simulink model "CodeGenValidation"  (R2018b)
settings: Solver=FixedStepDiscrete  StartTime=0.0  StopTime=60  FixedStep=MdlTS  RelTol=1e-3  EnableMultiTasking=on
undefined symbols (not defined in the file or in its folder): sigbuilder_block
settings Model: DataDictionary=CodeGenPlantData.sldd  Creator=BRAUL  LastModifiedBy=BRAUL
settings OptimizationCC: DefaultParameterBehavior=Inlined  UseFloatMulNetSlope=on  UseSpecifiedMinMax=on  InlineInvariantSignals=on  PassReuseOutputArgsAs=Individual arguments  ZeroExternalMemoryAtStartup=off  ZeroInternalMemoryAtStartup=off  NoFixptDivByZeroProtection=on  EfficientFloat2IntCast=on  LifeSpan=inf  MaxStackSize=64  OptimizeBlockOrder=speed  DifferentSizesBufferReuse=on
settings DebuggingCC: MergeDetectMultiDrivingBlocksExec=none  ParameterTunabilityLossMsg=error
settings HardwareCC: ProdBitPerPointer=32  ProdBitPerSizeT=32  ProdBitPerPtrDiffT=32  ProdLargestAtomicInteger=Long  ProdLargestAtomicFloat=Double  ProdWordSize=32  ProdLongLongMode=on  ProdHWDeviceType=ARM Compatible->ARM Cortex
settings ModelReferenceCC: ModelReferenceNumInstancesAllowed=Single  PropagateSignalLabelsOutOfModel=off
settings SFSimCC: MATLABDynamicMemAlloc=off
settings RTWCC: SystemTargetFile=ert.tlc  HardwareBoard=STM32 Nucleo F411RE  TemplateMakefile=ert_default_tmf  GenerateReport=on  Toolchain=GNU Tools for ARM Embedded Processors  BuildConfiguration=Faster Runs  IncludeHyperlinkInReport=on  LaunchReport=on  CodeExecutionProfiling=on  GenerateTraceInfo=on  GenerateTraceReport=on  GenerateTraceReportSl=on  GenerateTraceReportSf=on  GenerateTraceReportEml=on
settings CodeAppCC: ForceParamTrailComments=on  IgnoreCustomStorageClasses=off  OperatorAnnotations=on  SimulinkDataObjDesc=on  SFDataObjDesc=on  InsertBlockDesc=on
settings ERTTargetCC: CombineSignalStateStructs=on  SuppressErrorStatus=on  SupportNonFinite=off  SupportComplex=off

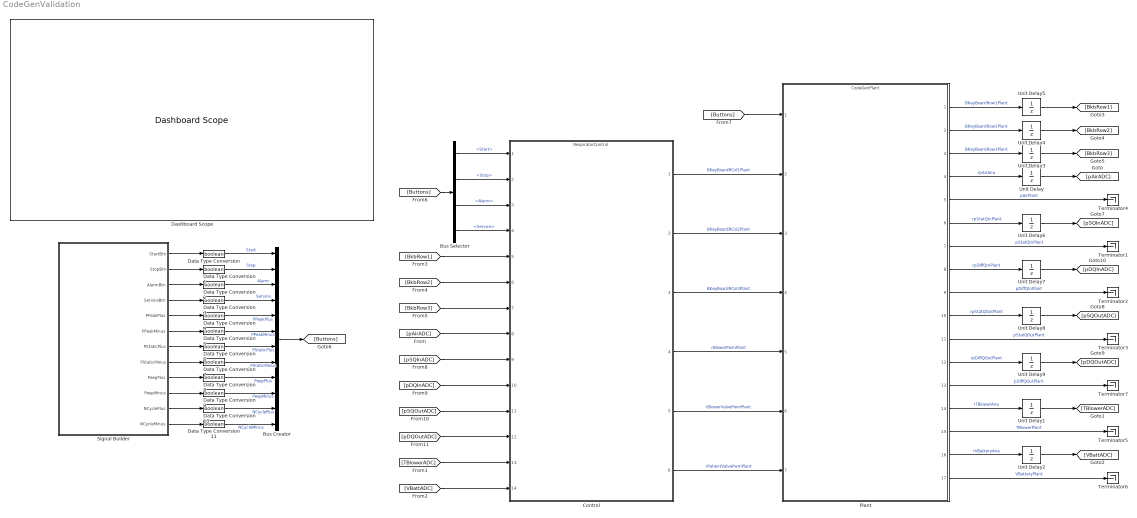
== system CodeGenValidation ==
  Bus Creator : BusCreator  Inputs=12  OutDataTypeStr=Bus: UserButtons
  Bus Selector : BusSelector  OutputSignals=Start,Stop,Alarm,Service
  Control : ModelReference  ModelNameDialog=RespiratorControl.slx  SimulationMode=Processor-in-the-loop (PIL)  ModelReferenceVersion=1.242
  Dashboard Scope : DashboardScope  WebBlockId=143  Ymin=0  Ymax=500
  Data Type Conversion{,1..11} (12 alike) : DataTypeConversion  OutDataTypeStr=boolean
  Plant : ModelReference  ModelNameDialog=CodeGenPlant.slx  SimulationMode=Normal  ModelReferenceVersion=1.68
  Signal Builder : Subsystem  Tag=STV Subsys  LoadFcn=sigbuilder_block('load');  StartFcn=sigbuilder_block('start');  StopFcn=sigbuilder_block('stop');  ClipboardFcn=sigbuilder_block('clipboard');  mask(Sigbuilder block){tuvar=[0:10]}
      mask help: Simulink:masks:SigbuilderBlock_MD
      mask init:
      | if ~strcmp(get_param(bdroot(gcbh),'SimulationStatus'),'stopped') tuvar = sigbuilder_block('maskInit'); end
      settings: CopyFcn=sigbuilder_block('copy');  DeleteFcn=sigbuilder_block('delete');  ModelCloseFcn=sigbuilder_block('modelClose');  PreSaveFcn=sigbuilder_block('preSave');  PauseFcn=sigbuilder_block('pause');  ContinueFcn=sigbuilder_block('continue');  NameChangeFcn=sigbuilder_block('namechange');  OpenFcn=sigbuilder_block('open',[6 0 1428 711.75 ]);  CloseFcn=sigbuilder_block('close');
      mask Display: plot(0, 0, 100, 100,[2, 2, 32, 32, 2], [68, 8, 8, 68, 68],[32, 2], [38, 38], [32, 19, 2],[53, 60, 44], [32, 17, 17, 2],[16, 16, 31, 31]);txt = getActiveGroup(gcbh);text(2, 100, txt,'verticalAlignment', 'top');
  Terminator{1..7} (7 alike) : Terminator
  Unit Delay{,2..5} (5 alike) : UnitDelay  SampleTime=-1
  Unit Delay{1,6..9} (5 alike) : UnitDelay  InitialCondition=0.7619  SampleTime=-1
  wires:
  Control/4 -> Plant/5  "rBlowerPwmPlant"
  Control/5 -> Plant/6  "rBlowerValvePwmPlant"
  Control/6 -> Plant/7  "rPatientValvePwmPlant"
  Plant/4 -> Unit Delay/1  "rpAirAna"
  Unit Delay/1 -> [pAirADC]
  [pAirADC] -> Control/8
  Bus Selector/1 -> Control/1  "<Start>"
  Bus Selector/2 -> Control/2  "<Stop>"
  Bus Selector/3 -> Control/3  "<Alarm>"
  Bus Selector/4 -> Control/4  "<Service>"
  Plant/5 -> Terminator4/1  "pAirPlant"
  Plant/15 -> Terminator5/1  "TBlowerPlant"
  Plant/17 -> Terminator6/1  "VBatteryPlant"
  Unit Delay1/1 -> [TBlowerADC]
  Plant/14 -> Unit Delay1/1  "rTBlowerAna"
  Plant/16 -> Unit Delay2/1  "rVBatteryAna"
  Unit Delay2/1 -> [VBattADC]
  [VBattADC] -> Control/14
  [TBlowerADC] -> Control/13
  Control/3 -> Plant/4  "BKeyBoardRCol3Plant"
  Control/2 -> Plant/3  "BKeyBoardRCol2Plant"
  Control/1 -> Plant/2  "BKeyBoardRCol1Plant"
  Plant/1 -> Unit Delay5/1  "BKeyBoardRow1Plant"
  Plant/2 -> Unit Delay4/1  "BKeyBoardRow2Plant"
  Plant/3 -> Unit Delay3/1  "BKeyBoardRow3Plant"
  Unit Delay5/1 -> [BkbRow1]
  Unit Delay4/1 -> [BkbRow2]
  Unit Delay3/1 -> [BkbRow3]
  [BkbRow1] -> Control/5
  [BkbRow2] -> Control/6
  [BkbRow3] -> Control/7
  Signal Builder/1(StartBtn) -> Data Type Conversion/1
  Signal Builder/2(StopBtn) -> Data Type Conversion1/1
  Signal Builder/3(AlarmBtn) -> Data Type Conversion2/1
  Signal Builder/4(ServiceBtn) -> Data Type Conversion3/1
  Signal Builder/5(PPeakPlus) -> Data Type Conversion4/1
  Signal Builder/6(PPeakMinus) -> Data Type Conversion5/1
  Signal Builder/7(PStaticPlus) -> Data Type Conversion6/1
  Signal Builder/8(PStaticMinus) -> Data Type Conversion7/1
  Signal Builder/9(PeepPlus) -> Data Type Conversion8/1
  Signal Builder/10(PeepMinus) -> Data Type Conversion9/1
  Signal Builder/11(NCyclePlus) -> Data Type Conversion10/1
  Signal Builder/12(NCycleMinus) -> Data Type Conversion11/1
  Bus Creator/1 -> [Buttons]
  [Buttons] -> Bus Selector/1
  [Buttons] -> Plant/1
  Data Type Conversion/1 -> Bus Creator/1  "Start"
  Data Type Conversion1/1 -> Bus Creator/2  "Stop"
  Data Type Conversion2/1 -> Bus Creator/3  "Alarm"
  Data Type Conversion3/1 -> Bus Creator/4  "Service"
  Data Type Conversion4/1 -> Bus Creator/5  "PPeakPlus"
  Data Type Conversion5/1 -> Bus Creator/6  "PPeakMinus"
  Data Type Conversion6/1 -> Bus Creator/7  "PStaticPlus"
  Data Type Conversion7/1 -> Bus Creator/8  "PStaticMinus"
  Data Type Conversion8/1 -> Bus Creator/9  "PeepPlus"
  Data Type Conversion9/1 -> Bus Creator/10  "PeepMinus"
  Data Type Conversion10/1 -> Bus Creator/11  "NCyclePlus"
  Data Type Conversion11/1 -> Bus Creator/12  "NCycleMinus"
  Plant/7 -> Terminator1/1  "pStatQInPlant"
  Plant/9 -> Terminator2/1  "pDiffQInPlant"
  Plant/11 -> Terminator3/1  "pStatQOutPlant"
  Plant/13 -> Terminator7/1  "pDiffQOutPlant"
  Plant/6 -> Unit Delay6/1  "rpStatQInPlant"
  Plant/10 -> Unit Delay8/1  "rpStatQOutPlant"
  Plant/8 -> Unit Delay7/1  "rpDiffQInPlant"
  Plant/12 -> Unit Delay9/1  "rpDiffQOutPlant"
  Unit Delay6/1 -> [pSQInADC]
  Unit Delay8/1 -> [pSQOutADC]
  Unit Delay9/1 -> [pDQOutADC]
  Unit Delay7/1 -> [pDQInADC]
  [pSQInADC] -> Control/9
  [pDQInADC] -> Control/10
  [pSQOutADC] -> Control/11
  [pDQOutADC] -> Control/12

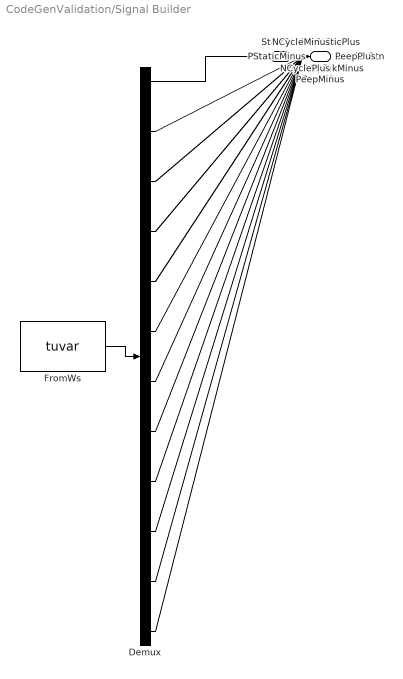
== system CodeGenValidation/Signal Builder ==
  Demux : Demux  Tag=STV Demux  Outputs=12
  FromWs : FromWorkspace  Tag=STV FromWs  VariableName=tuvar  SampleTime=0
      SigBuilderData=|
      | common.afterFinalStr = 'Extrapolate'
      | common.sampleTime = 0
      | dataSet.timeRange = [0 60]
      | dataSet.name = 'Group 1'
      | sbobj.Groups.Name = 'Group 1'
      | sbobj.Groups.Signals(1).Name = 'StartBtn'
      | sbobj.Groups.Signals(1).XData = [0 2 2 2.113 2.113 3 3 3.3 3.3 5.4 5.4 5.65 5.65 14 16 18 20 22 24 26 28 30 32 34 36 38 40 42 44 46 48 50 52 54 56 59.4 59.4 60]
      | sbobj.Groups.Signals(1).YData = [0 0 1 1 0 0 1 1 0 0 1 1 0 0 0 0 0 0 0 0 0 0 0 0 0 0 0 0 0 0 0 0 0 0 0 0 1 1]
      | sbobj.Groups.Signals(2).Name = 'StopBtn'
      | sbobj.Groups.Signals(2).XData = [0 0.75 0.75 1.1 1.1 6 8 10 12 14 16 18 20 22 24 26 28 30 32 34 36 38 40 42 44 46 48 56.05 56.05 56.07 56.07 57.1 57.1 57.65 57.65 58 60]
      | sbobj.Groups.Signals(2).YData = [0 0 1 1 0 0 0 0 0 0 0 0 0 0 0 0 0 0 0 0 0 0 0 0 0 0 0 0 1 1 0 0 1 1 0 0 0]
      | sbobj.Groups.Signals(3).Name = 'AlarmBtn'
      | sbobj.Groups.Signals(3).XData = [0 2 4 6 8 10 12 14 16 18 20 22 24 26 26 26.3 26.3 30 32 34 36 38 40 43.75 43.75 44 44 46 48 50 52 54 54 54.1 54.1 58 60]
      | sbobj.Groups.Signals(3).YData = [0 0 0 0 0 0 0 0 0 0 0 0 0 0 1 1 0 0 0 0 0 0 0 0 1 1 0 0 0 0 0 0 1 1 0 0 0]
      | sbobj.Groups.Signals(4).Name = 'ServiceBtn'
      | sbobj.Groups.Signals(4).XData = [0 2 4 6 8 10 12 14 16 18 20 22 24 26 28 30 32 34 36 38 40 40.7 40.7 41.2 41.2 46 48 50 52 54 56 58 60]
      | sbobj.Groups.Signals(4).YData = [0 0 0 0 0 0 0 0 0 0 0 0 0 0 0 0 0 0 0 0 0 0 1 1 0 0 0 0 0 0 0 0 0]
      | sbobj.Groups.Signals(5).Name = 'PPeakPlus'
      | sbobj.Groups.Signals(5).XData = [0 10.75 10.75 11 11 11.8 11.8 12.15 12.15 13.05 13.05 13.3 13.3 14.1 14.1 14.45 14.45 18 20 22 24 26 28 30 32 34 36 38 40 42 44 46 48 50 52 54 56 58 60]
      | sbobj.Groups.Signals(5).YData = [0 0 1 1 0 0 1 1 0 0 1 1 0 0 1 1 0 0 0 0 0 0 0 0 0 0 0 0 0 0 0 0 0 0 0 0 0 0 0]
      | sbobj.Groups.Signals(6).Name = 'PPeakMinus'
      | sbobj.Groups.Signals(6).XData = [0 15.55 17.4 18.25 18.25 18.65 18.65 19.35 19.35 19.7 19.7 20.2 20.2 20.245 20.245 21.3 21.3 21.6 21.6 22 24 26 28 30 32 34 36 38 38 38.2 38.2 42 44 46 48 50 52 54 56 58 60]
      | sbobj.Groups.Signals(6).YData = [0 0 0 0 1 1 0 0 1 1 0 0 1 1 0 0 1 1 0 0 0 0 0 0 0 0 0 0 1 1 0 0 0 0 0 0 0 0 0 0 0]
      | sbobj.Groups.Signals(7).Name = 'PStaticPlus'
      | sbobj.Groups.Signals(7).XData = [0 2 4 6 8 10 12 14 16 18 20 22 24 30.4 30.4 30.8 30.8 31.65 31.65 32 32 32.85 32.85 33.25 33.25 34.1 34.1 34.35 34.35 34.8 34.8 34.819 34.819 46 48 50 52 54 56 58 60]
      | sbobj.Groups.Signals(7).YData = [0 0 0 0 0 0 0 0 0 0 0 0 0 0 1 1 0 0 1 1 0 0 1 1 0 0 1 1 0 0 1 1 0 0 0 0 0 0 0 0 0]
      | sbobj.Groups.Signals(8).Name = 'PStaticMinus'
      | sbobj.Groups.Signals(8).XData = [0 2 4 6 8 10 12 14 16 18 20 22 24 26 28 30.4 30.4 30.8 30.8 38.45 38.45 38.8 38.8 39.7 39.7 40 40 40.5 40.5 40.65 40.65 41.55 41.55 41.85 41.85 42.3 42.3 42.6 42.6 54 56 58 60]
      | sbobj.Groups.Signals(8).YData = [0 0 0 0 0 0 0 0 0 0 0 0 0 0 0 0 1 1 0 0 1 1 0 0 1 1 0 0 1 1 0 0 1 1 0 0 1 1 0 0 0 0 0]
      | sbobj.Groups.Signals(9).Name = 'PeepPlus'
      | sbobj.Groups.Signals(9).XData = [0 2 4 6 8 10.95 10.95 11.3 11.3 14 16 16.6 16.6 16.85 16.85 23.7 23.7 24 24 25 25 25.3 25.3 30 32 34 36 38 40 42 44 49.05 49.05 49.35 49.35 50 50 50.25 50.25 54 56 58 60]
      | sbobj.Groups.Signals(9).YData = [0 0 0 0 0 0 1 1 0 0 0 0 1 1 0 0 1 1 0 0 1 1 0 0 0 0 0 0 0 0 0 0 1 1 0 0 1 1 0 0 0 0 0]
      | sbobj.Groups.Signals(10).Name = 'PeepMinus'
      | sbobj.Groups.Signals(10).XData = [0 2 2 2.35 2.35 6 6 6.3 6.3 8.9 8.9 9.15 9.15 14.75 14.75 15.15 15.15 18 20 22 24 26 28 30 32 34 36 38 40 42 44 46 46 46.25 46.25 52.95 52.95 53.25 53.25 54 56 58 60]
      | sbobj.Groups.Signals(10).YData = [0 0 1 1 0 0 1 1 0 0 1 1 0 0 1 1 0 0 0 0 0 0 0 0 0 0 0 0 0 0 0 0 1 1 0 0 1 1 0 0 0 0 0]
      | sbobj.Groups.Signals(11).Name = 'NCyclePlus'
      | sbobj.Groups.Signals(11).XData = [0 2 4 6 8 10 12 14 16 18 20 22 24 27.7 27.7 28 28 30 32 36.65 36.65 36.95 36.95 38 40 42 44 47.55 47.55 48 48 50 52 54 56 58 60]
      | sbobj.Groups.Signals(11).YData = [0 0 0 0 0 0 0 0 0 0 0 0 0 0 1 1 0 0 0 0 1 1 0 0 0 0 0 0 1 1 0 0 0 0 0 0 0]
      | sbobj.Groups.Signals(12).Name = 'NCycleMinus'
      | sbobj.Groups.Signals(12).XData = [0 3.75 3.75 4 4 6 8 10 12 16.75 16.75 17 17 18 18 18.3 18.3 22 24 26 28 30 30 30.35 30.35 34 36 39.7 39.7 40 40 42 44 46 48 51.75 51.75 52 52 54 56 58 60]
      | sbobj.Groups.Signals(12).YData = [0 0 1 1 0 0 0 0 0 0 1 1 0 0 1 1 0 0 0 0 0 0 1 1 0 0 0 0 1 1 0 0 0 0 0 0 1 1 0 0 0 0 0]
      | sbobj.Groups.TimeRange = [0 60]
  StartBtn : Outport  Tag=STV Outport
  StopBtn : Outport  Tag=STV Outport  Port=2
  AlarmBtn : Outport  Tag=STV Outport  Port=3
  ServiceBtn : Outport  Tag=STV Outport  Port=4
  PPeakPlus : Outport  Tag=STV Outport  Port=5
  PPeakMinus : Outport  Tag=STV Outport  Port=6
  PStaticPlus : Outport  Tag=STV Outport  Port=7
  PStaticMinus : Outport  Tag=STV Outport  Port=8
  PeepPlus : Outport  Tag=STV Outport  Port=9
  PeepMinus : Outport  Tag=STV Outport  Port=10
  NCyclePlus : Outport  Tag=STV Outport  Port=11
  NCycleMinus : Outport  Tag=STV Outport  Port=12
  wires:
  Demux/1 -> StartBtn/1
  FromWs/1 -> Demux/1
  Demux/2 -> StopBtn/1
  Demux/3 -> AlarmBtn/1
  Demux/4 -> ServiceBtn/1
  Demux/5 -> PPeakPlus/1
  Demux/6 -> PPeakMinus/1
  Demux/7 -> PStaticPlus/1
  Demux/8 -> PStaticMinus/1
  Demux/9 -> PeepPlus/1
  Demux/10 -> PeepMinus/1
  Demux/11 -> NCyclePlus/1
  Demux/12 -> NCycleMinus/1
